simulink model "Final_FCcontrol"  (R2023a)
settings: Solver=VariableStepAuto  StartTime=0.0  StopTime=22  RelTol=1e-3
undefined symbols (not defined in the file): I_P_TLU
settings Model: Creator=Abhinandan  LastModifiedBy=Abhinandan

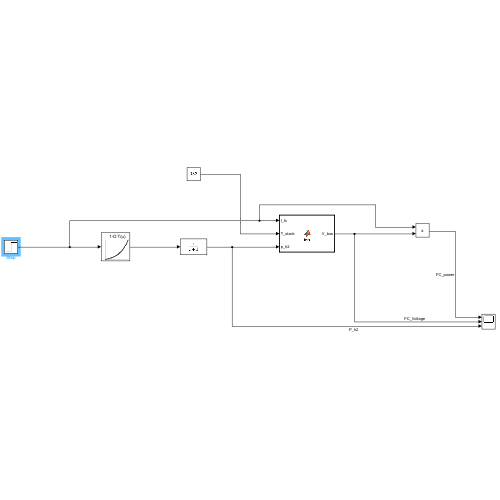
[thumbnail: Simulink's stored preview of the top-level diagram]
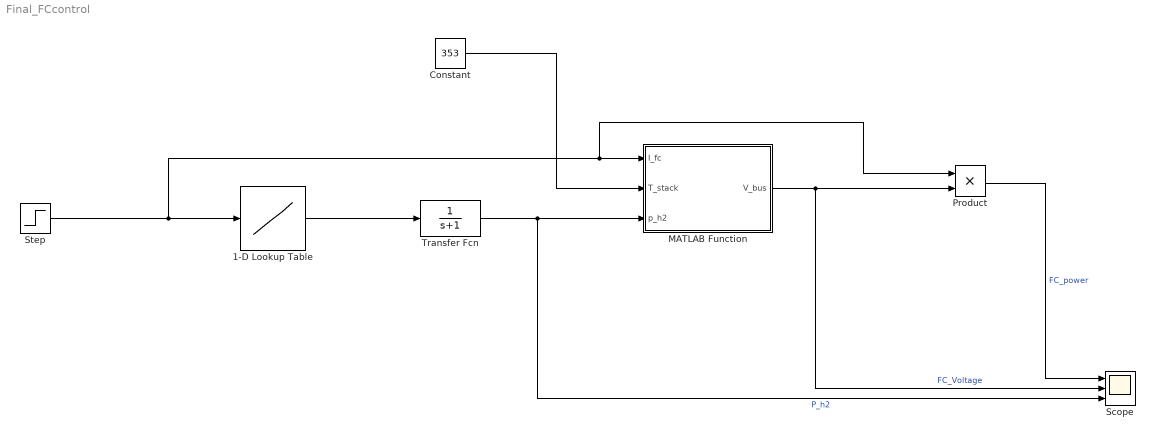
== system Final_FCcontrol ==
  1-D Lookup Table : Lookup_n-D  NumberOfTableDimensions=1  BreakpointsForDimension1=I_P_TLU.Current  Table=I_P_TLU.Pressure  InternalRulePriority=Speed  RndMeth=Simplest
  Constant : Constant  Value=353
  MATLAB Function : MATLAB Function  TreatAsAtomicUnit=on
  Product : Product
  Scope : Scope  NumInputPorts=3
  Step : Step  Time=15  Before=107  After=154  SampleTime=0
  Transfer Fcn : TransferFcn  Denominator=[1 1]
  wires:
  1-D Lookup Table/1 -> Transfer Fcn/1
  Transfer Fcn/1 -> Scope/3, MATLAB Function/3(p_h2)  "P_h2"
  Constant/1 -> MATLAB Function/2(T_stack)
  MATLAB Function/1(V_bus) -> Scope/2, Product/2  "FC_Voltage"
  Product/1 -> Scope/1  "FC_power"
  Step/1 -> 1-D Lookup Table/1, Product/1, MATLAB Function/1(I_fc)

== matlab function Final_FCcontrol/MATLAB Function ==
  data: I_fc input; T_stack input; p_h2 input; V_bus output
function V_bus = fcn(I_fc,T_stack,p_h2)                %T_stack in K, T_fc in A, V_bus in V
    F = 96485.33;       
    R = 8.31447;
    i_lim = 1.4;
    A_cell = 500;
    N_cell = 300;

    E_cell = -237.14e+3/(-2*F);
    i_cell = I_fc/A_cell;
    
    i0 = 8e-05;
    alpha = 0.5;
    t_membrane = 125e-4;
    
    a = 0.5;
    lambda_m = 0.043 + 17.81*a - 39.85*a^2 + 36*a^3;
    sigma_30 = 0.005139*lambda_m - 0.00326;
    sigma = sigma_30*exp(1268*(1/303.15 - 1/T_stack));
    
    b = (R*T_stack)/(2*alpha*F);  

    V_nernst = E_cell + R*T_stack/(2*F) * log((3/4)^(1/2)*p_h2^(3/2));

    V_act = b*log(i_cell/i0);

    R_ohm = t_membrane/sigma;
    V_ohm = i_cell*R_ohm;

    V_conc = -R*T_stack/(2*F) * log(1-(i_cell/i_lim));          
    V_cell = V_nernst - V_act - V_ohm - V_conc;


    V_bus = V_cell*N_cell;
end
